simulink model "model"  (R2022b)
settings: Solver=VariableStepAuto  StartTime=0.0  StopTime=3  FixedStep=Tsi/10  RelTol=2e-4
undefined symbols (not defined in the file): B, B0, Hpp, Imax, In, Kdp_si, Ke, Kf, Ki_si, Kip_si, Kp_si, Kpp_si, Kppph_si, Kpppl_si, L, M, max_ppa_si, max_ppv_si, R, Umax
libraries: simulink x3, slctrlblks x1
settings Model: Creator=Giulio  LastModifiedBy=niczan1
settings DebuggingCC: UnconnectedInputMsg=warning  UnconnectedOutputMsg=warning  UnconnectedLineMsg=warning  SFMachineParentedDataDiag=warning
settings ModelReferenceCC: EnableRefExpFcnMdlSchedulingChecks=on

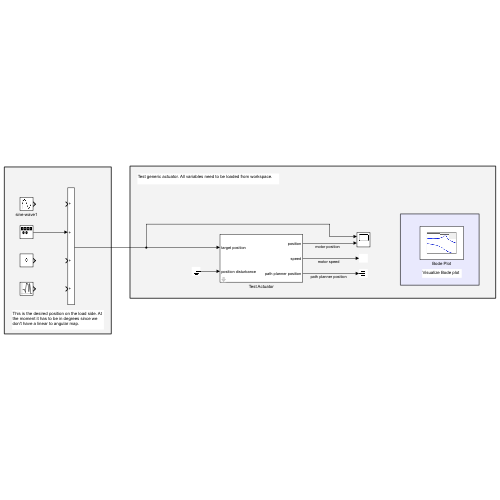
[thumbnail: Simulink's stored preview of the top-level diagram]
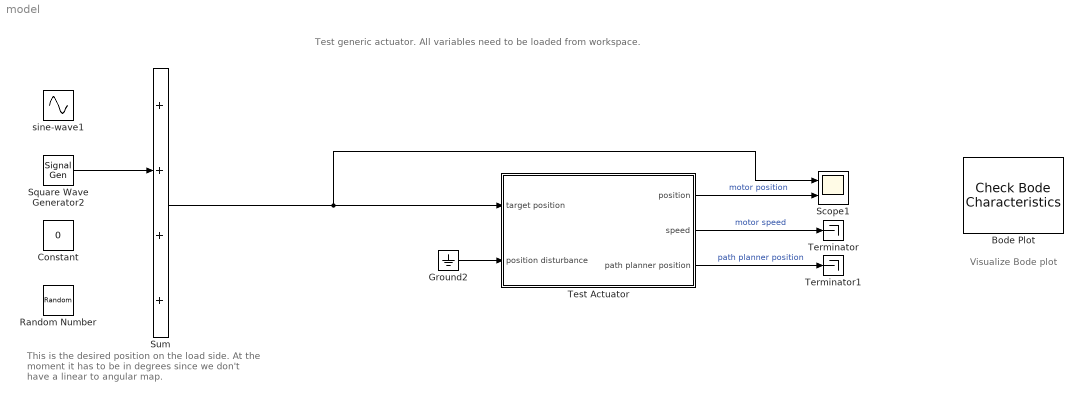
== system model ==
  note: This is the desired position on the load side. At the moment it has to be in degrees since we don't have a linear to angular map.
  note: Visualize Bode plot
  note: Test generic actuator. All variables need to be loaded from workspace.
  Bode Plot : slctrlblks/Model Verification/Check Bode  Characteristics  InstantiateOnLoad=on  SaveOperatingPoints=off  LinearizationIOs={'/Sum', 1, 'in', 'off', '';'/Test Actuator', 1, 'out', 'on', ''}  LinearizeAt=SnapshotTimes  SnapshotTimes=[0]  TriggerType=rising  SampleTime=auto  RateConversionMethod=zoh  PreWarpFreq=10  UseExactDelayModel=off  UseFullBlockNameLabels=off  UseBusSignalLabels=off  enabled=on  stopWhenAssertionFail=off  export=off  ViewDlgPos=[2544 169 510 390]  OpenViewOnLoad=off  LaunchViewOnOpen=on  FrequencyUnits=rad/s  MagnitudeUnits=dB  PhaseUnits=deg  TimeUnits=seconds  EnableUpperBound=off  UpperBoundFrequencies=[]  UpperBoundMagnitudes=[]  EnableLowerBound=off  LowerBoundFrequencies=[]  LowerBoundMagnitudes=[]
      settings: LibrarySourceBlock=slctrlblks/Linear Analysis Plots/Bode Plot
  Constant : Constant  Value=0
  Ground2 : Ground
  Random Number : RandomNumber  Variance=1e-10  SampleTime=1e-3
  Scope1 : Scope  NumInputPorts=2
  Square Wave Generator2 : SignalGenerator  WaveForm=square  Amplitude=15e-3
  Sum : Sum  Inputs=++++
  Terminator : Terminator
  Terminator1 : Terminator
  Test Actuator : Subsystem  mask(Motor servo){Tsi=4e-5, Tsp=4e-4, Tspp=4e-4}
      mask DialogControl SamplingTimes Prompt: Sampling times
  sine-wave1 : Sin  Amplitude=2.5e-3  Frequency=2*pi*4  SampleTime=0
  wires:
  Sum/1 -> Test Actuator/1(target position), Scope1/1
  Test Actuator/3(path planner position) -> Terminator1/1  "path planner position"
  Test Actuator/2(speed) -> Terminator/1  "motor speed"
  Ground2/1 -> Test Actuator/2(position disturbance)
  Square Wave Generator2/1 -> Sum/2
  Test Actuator/1(position) -> Scope1/2  "motor position"

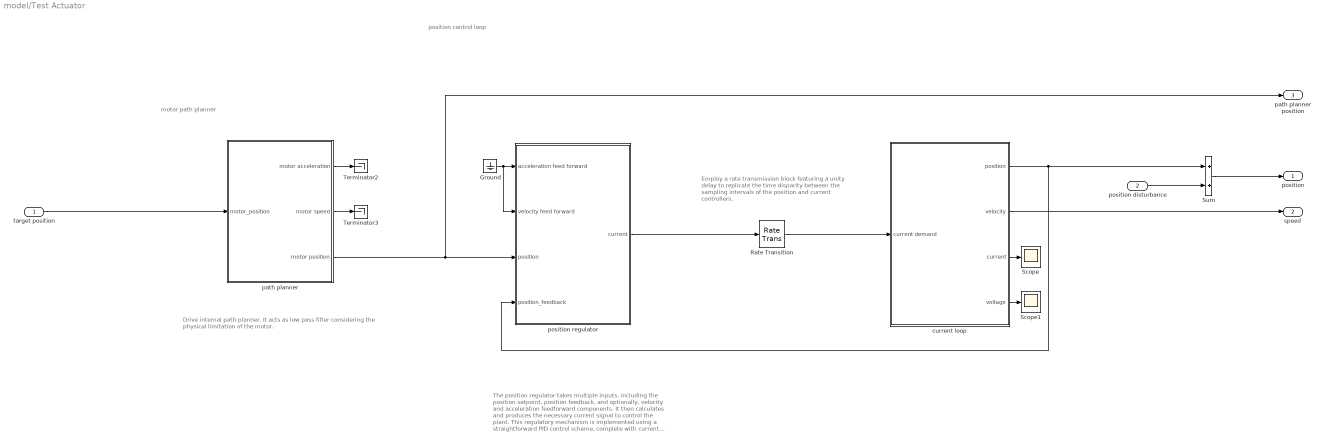
== system model/Test Actuator ==
  note: position control loop
  note: Employ a rate transmission block featuring a unity delay to replicate the time disparity between the sampling intervals of the position and current controllers.
  note: The position regulator takes multiple inputs, including the position setpoint, position feedback, and optionally, velocity and acceleration feedforward components. It then calculates and produces the necessary current signal to control the plant. This regulatory mechanism is implemented using a straightforward PID control scheme, complete with current saturation (limited to the motor's nominal current) and anti-windup provisions.
  note: motor path planner
  note: Drive internal path planner. It acts as low pass filter considering the physical limitation of the motor.
  target position : Inport
  position disturbance : Inport  Port=2
  Ground : Ground
  Rate Transition : RateTransition
  Scope : Scope
  Scope1 : Scope
  Sum : Sum
  Terminator2 : Terminator
  Terminator3 : Terminator
  current loop : Subsystem
  path planner : Subsystem  TreatAsAtomicUnit=on  SystemSampleTime=Tspp  mask(Drive internal path planner){Active=off, max_ppa_si=max_ppa_si, max_ppv_si=max_ppv_si, Kppph_si=Kppph_si, Kpppl_si=Kpppl_si, Hpp=Hpp}
      mask prompts: max_ppa_si "Max acceleration"; max_ppv_si "Max speed"; Kppph_si "High gain"; Kpppl_si "Low gain"; Hpp "Exponential"
      mask DialogControl ParameterGroupVar Prompt: Status
      mask DialogControl Container3 Prompt: Saturation
      mask DialogControl Container4 Prompt: Controller
  position regulator : Subsystem  TreatAsAtomicUnit=on  SystemSampleTime=Tsp  mask(Position PID controller){In=In, Imax=Imax, Kpp_si=Kpp_si, Kip_si=Kip_si, Kdp_si=Kdp_si, FF_w_si=0, FF_a_si=0}
      mask prompts: In "Nominal current"; Imax "Max current"; Kpp_si "Proportional gain"; Kip_si "Integral gain"; Kdp_si "Derivative gain"; FF_w_si "Velocity feed forward gain"; FF_a_si "Acceleration feed forward gain"
      mask DialogControl Saturation Prompt: Saturation
      mask DialogControl Controller Prompt: Controller
  position : Outport
  speed : Outport  Port=2
  path planner position : Outport  Port=3
  wires:
  position regulator/1(current) -> Rate Transition/1
  current loop/1(position) -> Sum/1, position regulator/4(position_feedback)
  Rate Transition/1 -> current loop/1(current demand)
  current loop/4(voltage) -> Scope1/1
  current loop/3(current) -> Scope/1
  path planner/2(motor speed) -> Terminator3/1
  path planner/1(motor acceleration) -> Terminator2/1
  Ground/1 -> position regulator/2(velocity feed forward), position regulator/1(acceleration feed forward)
  target position/1 -> path planner/1(motor_position)
  current loop/2(velocity) -> speed/1
  position disturbance/1 -> Sum/2
  Sum/1 -> position/1
  path planner/3(motor position) -> path planner position/1, position regulator/3(position)

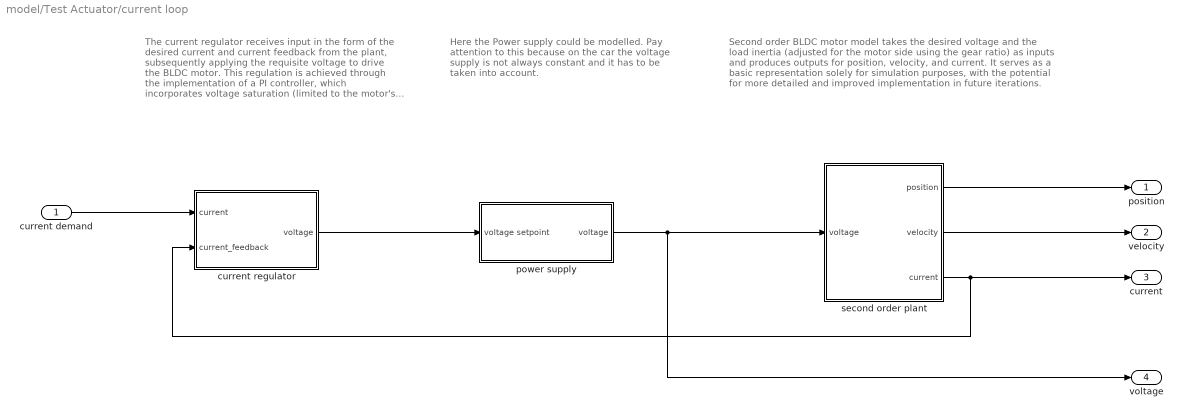
== system model/Test Actuator/current loop ==
  note: The current regulator receives input in the form of the desired current and current feedback from the plant, subsequently applying the requisite voltage to drive the BLDC motor. This regulation is achieved through the implementation of a PI controller, which incorporates voltage saturation (limited to the motor's nominal voltage) and anti-windup mechanisms.
  note: Second order BLDC motor model takes the desired voltage and the load inertia (adjusted for the motor side using the gear ratio) as inputs and produces outputs for position, velocity, and current. It serves as a basic representation solely for simulation purposes, with the potential for more detailed and improved implementation in future iterations.
  note: Here the Power supply could be modelled. Pay attention to this because on the car the voltage supply is not always constant and it has to be taken into account.
  current demand : Inport
  current regulator : Subsystem  TreatAsAtomicUnit=on  SystemSampleTime=Tsi  mask(Current PI controller){Umax=Umax, Un=Umax, Kp_si=Kp_si, Ki_si=Ki_si}
      mask prompts: Umax "Max voltage"; Un "Nominal voltage"; Kp_si "Proportional gain"; Ki_si "Integral gain"
      mask DialogControl Saturation Prompt: Saturation
      mask DialogControl Controller Prompt: Controller
  power supply : Subsystem
  second order plant : Subsystem  mask(Motor second order model){Ke=Ke, R=R, L=L, Kf=Kf, M=M, B=B, B0=B0}
      mask prompts: Ke "Electrical constant"; R "Resistance"; L "Inductance"; Kf "Force constant"; M "Motor mass"; B "Viscous friction"; B0 "Static friction"
      mask DialogControl electrical Prompt: Electrical
      mask DialogControl Mechanical Prompt: Mechanical
  position : Outport
  velocity : Outport  Port=2
  current : Outport  Port=3
  voltage : Outport  Port=4
  wires:
  second order plant/2(velocity) -> velocity/1
  current demand/1 -> current regulator/1(current)
  second order plant/1(position) -> position/1
  second order plant/3(current) -> current regulator/2(current_feedback), current/1
  power supply/1(voltage) -> second order plant/1(voltage), voltage/1
  current regulator/1(voltage) -> power supply/1(voltage setpoint)

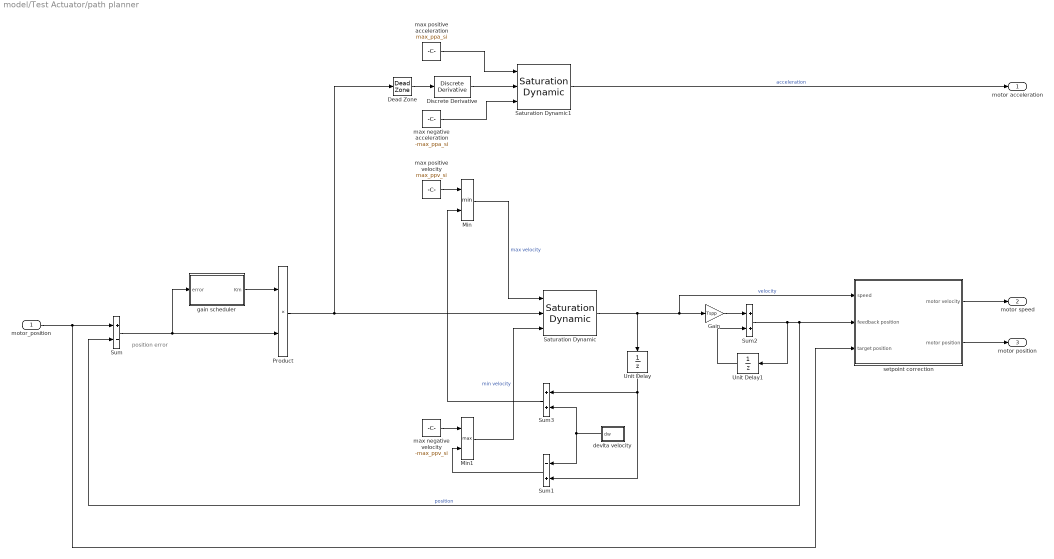
== system model/Test Actuator/path planner ==
  note: position error
  motor_position : Inport
  Dead Zone : DeadZone  LowerValue=-0.01  UpperValue=0.01
  Discrete Derivative : simulink/Discrete/Discrete Derivative  gainval=1.0  ICPrevScaledInput=0.0  OutMin=[]  OutMax=[]  OutDataType=fixdt(1, 16)  OutScaling=2^-10  DoSatur=off
  Gain : Gain  Gain=Tspp
  Min : MinMax  Inputs=2
  Min1 : MinMax  Function=max  Inputs=2
  Product : Product
  Saturation Dynamic : simulink/Discontinuities/Saturation Dynamic  OutMin=[]  OutMax=[]  OutDataTypeStr=Inherit: Same as second input  OutDataType=fixdt(1, 16)  OutScaling=2^-10  DoSatur=off
  Saturation Dynamic1 : simulink/Discontinuities/Saturation Dynamic  OutMin=[]  OutMax=[]  OutDataTypeStr=Inherit: Same as second input  OutDataType=fixdt(1, 16)  OutScaling=2^-10  DoSatur=off
  Sum : Sum  Inputs=+-
  Sum1 : Sum  Inputs=-+
  Sum2 : Sum
  Sum3 : Sum
  Unit Delay : UnitDelay  SampleTime=-1  HasFrameUpgradeWarning=on
  Unit Delay1 : UnitDelay  SampleTime=-1  HasFrameUpgradeWarning=on
  devlta velocity : Subsystem
  gain scheduler : Subsystem
  max negative acceleration : Constant  Value=-max_ppa_si
  max negative velocity : Constant  Value=-max_ppv_si
  max positive acceleration : Constant  Value=max_ppa_si
  max positive velocity : Constant  Value=max_ppv_si
  setpoint correction : Subsystem
  motor acceleration : Outport
  motor speed : Outport  Port=2
  motor position : Outport  Port=3
  wires:
  Sum/1 -> gain scheduler/1(error), Product/2
  max positive velocity/1 -> Min/1
  Saturation Dynamic/1 -> Gain/1, setpoint correction/1(speed), Unit Delay/1  "velocity"
  devlta velocity/1(dw) -> Sum1/1, Sum3/2
  Sum3/1 -> Min/2
  max negative velocity/1 -> Min1/1
  Sum1/1 -> Min1/2
  Min1/1 -> Saturation Dynamic/3  "min velocity"
  Min/1 -> Saturation Dynamic/1  "max velocity"
  Sum2/1 -> setpoint correction/2(feedback position), Sum/2, Unit Delay1/1  "position"
  Unit Delay/1 -> Sum3/1, Sum1/2
  max positive acceleration/1 -> Saturation Dynamic1/1
  max negative acceleration/1 -> Saturation Dynamic1/3
  Saturation Dynamic1/1 -> motor acceleration/1  "acceleration"
  Discrete Derivative/1 -> Saturation Dynamic1/2
  Dead Zone/1 -> Discrete Derivative/1
  setpoint correction/1(motor velocity) -> motor speed/1
  gain scheduler/1(Km) -> Product/1
  motor_position/1 -> setpoint correction/3(target position), Sum/1
  setpoint correction/2(motor position) -> motor position/1
  Product/1 -> Dead Zone/1, Saturation Dynamic/2
  Gain/1 -> Sum2/1
  Unit Delay1/1 -> Sum2/2

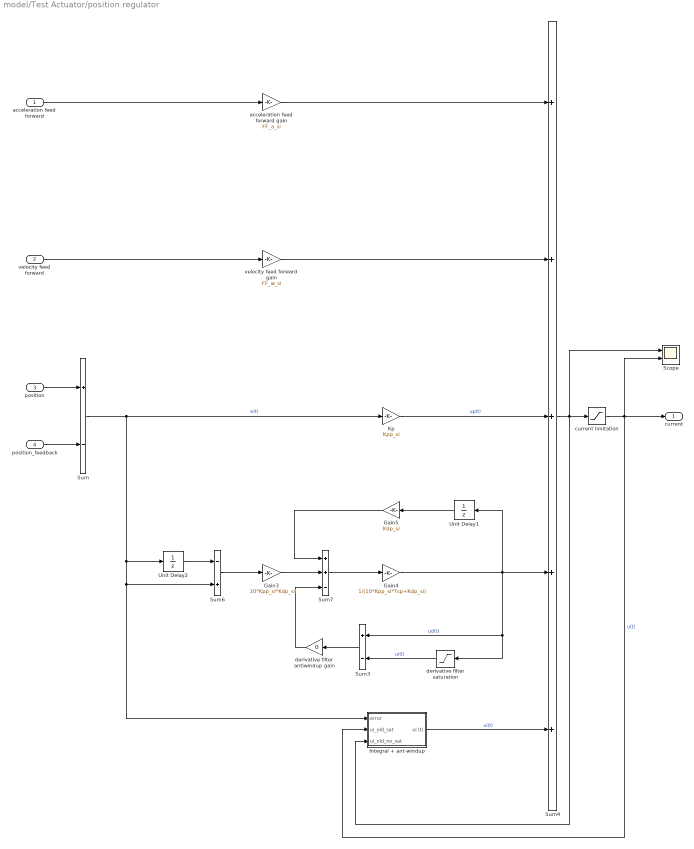
== system model/Test Actuator/position regulator ==
  acceleration feed forward : Inport
  velocity feed forward : Inport  Port=2
  position : Inport  Port=3
  position_feedback : Inport  Port=4
  Gain3 : Gain  Gain=10*Kpp_si*Kdp_si
  Gain4 : Gain  Gain=1/(10*Kpp_si*Tsp+Kdp_si)
  Gain5 : Gain  Gain=Kdp_si
  Integral + ant-windup : Subsystem
  Kp : Gain  Gain=Kpp_si
  Scope : Scope  NumInputPorts=2
  Sum : Sum  Inputs=+-
  Sum3 : Sum  Inputs=+-
  Sum4 : Sum  Inputs=+++++
  Sum6 : Sum  Inputs=-+
  Sum7 : Sum  Inputs=++-
  Unit Delay1 : UnitDelay  SampleTime=-1  HasFrameUpgradeWarning=on
  Unit Delay2 : UnitDelay  SampleTime=-1  HasFrameUpgradeWarning=on
  acceleration feed forward gain : Gain  Gain=FF_a_si
  current limitation : Saturate  UpperLimit=Imax  LowerLimit=-Imax
  derivative filter antiwindup gain : Gain  Gain=0
  derivative filter saturation : Saturate  UpperLimit=Imax/2  LowerLimit=-Imax/2
  velocity feed forward gain : Gain  Gain=FF_w_si
  current : Outport
  wires:
  acceleration feed forward gain/1 -> Sum4/1
  acceleration feed forward/1 -> acceleration feed forward gain/1
  velocity feed forward gain/1 -> Sum4/2
  velocity feed forward/1 -> velocity feed forward gain/1
  Sum7/1 -> Gain4/1
  current limitation/1 -> current/1, Scope/2, Integral + ant-windup/2(ui_old_sat)  "u(t)"
  Unit Delay2/1 -> Sum6/1
  Sum6/1 -> Gain3/1
  Unit Delay1/1 -> Gain5/1
  Kp/1 -> Sum4/3  "up(t)"
  Sum/1 -> Kp/1, Integral + ant-windup/1(error), Sum6/2, Unit Delay2/1  "e(t)"
  Gain3/1 -> Sum7/2
  Gain5/1 -> Sum7/1
  Gain4/1 -> Sum4/4, derivative filter saturation/1, Sum3/1, Unit Delay1/1  "ud(t)"
  Sum3/1 -> derivative filter antiwindup gain/1
  derivative filter saturation/1 -> Sum3/2  "ui(t)"
  derivative filter antiwindup gain/1 -> Sum7/3
  Integral + ant-windup/1(ui (t)) -> Sum4/5  "ui(t)"
  Sum4/1 -> Scope/1, current limitation/1, Integral + ant-windup/3(ui_old_no_sat)
  position/1 -> Sum/1
  position_feedback/1 -> Sum/2

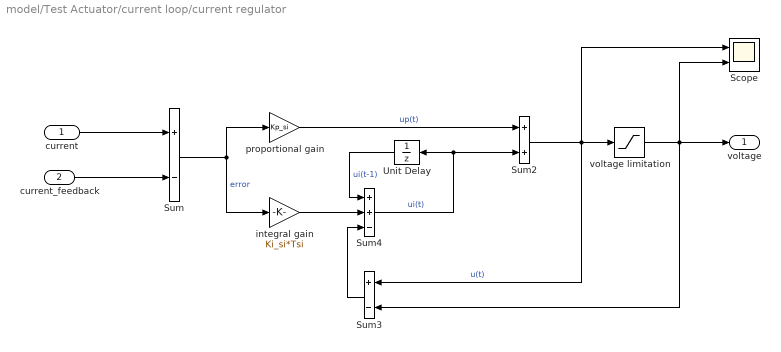
== system model/Test Actuator/current loop/current regulator ==
  current : Inport
  current_feedback : Inport  Port=2
  Scope : Scope  NumInputPorts=2
  Sum : Sum  Inputs=+-
  Sum2 : Sum
  Sum3 : Sum  Inputs=+-
  Sum4 : Sum  Inputs=++-
  Unit Delay : UnitDelay  SampleTime=-1  HasFrameUpgradeWarning=on
  integral gain : Gain  Gain=Ki_si*Tsi
  proportional gain : Gain  Gain=Kp_si
  voltage limitation : Saturate  UpperLimit=Umax  LowerLimit=-Umax
  voltage : Outport
  wires:
  voltage limitation/1 -> Scope/2, voltage/1, Sum3/2
  Sum3/1 -> Sum4/3
  Sum4/1 -> Unit Delay/1, Sum2/2  "ui(t)"
  Sum2/1 -> Sum3/1, Scope/1, voltage limitation/1  "u(t)"
  Sum/1 -> integral gain/1, proportional gain/1  "error"
  proportional gain/1 -> Sum2/1  "up(t)"
  current/1 -> Sum/1
  current_feedback/1 -> Sum/2
  Unit Delay/1 -> Sum4/1  "ui(t-1)"
  integral gain/1 -> Sum4/2

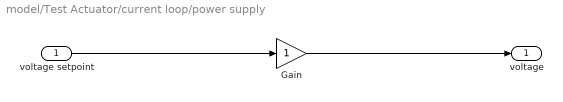
== system model/Test Actuator/current loop/power supply ==
  voltage setpoint : Inport
  Gain : Gain
  voltage : Outport
  wires:
  Gain/1 -> voltage/1
  voltage setpoint/1 -> Gain/1

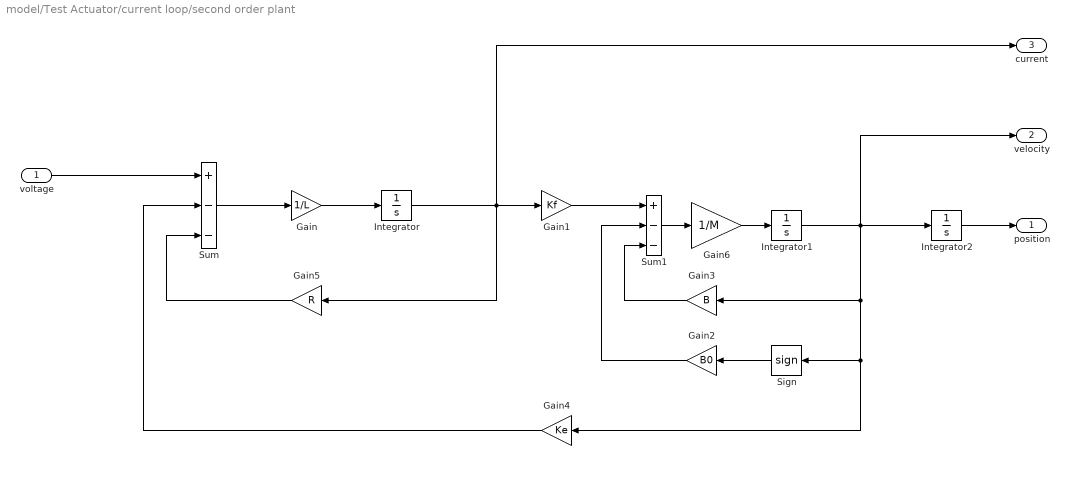
== system model/Test Actuator/current loop/second order plant ==
  voltage : Inport
  Gain : Gain  Gain=1/L
  Gain1 : Gain  Gain=Kf
  Gain2 : Gain  Gain=B0
  Gain3 : Gain  Gain=B
  Gain4 : Gain  Gain=Ke
  Gain5 : Gain  Gain=R
  Gain6 : Gain  Gain=1/M
  Integrator : Integrator
  Integrator1 : Integrator
  Integrator2 : Integrator
  Sign : Signum
  Sum : Sum  Inputs=+--
  Sum1 : Sum  Inputs=+--
  position : Outport
  velocity : Outport  Port=2
  current : Outport  Port=3
  wires:
  Integrator2/1 -> position/1
  voltage/1 -> Sum/1
  Gain/1 -> Integrator/1
  Sum1/1 -> Gain6/1
  Gain5/1 -> Sum/3
  Gain6/1 -> Integrator1/1
  Gain4/1 -> Sum/2
  Sum/1 -> Gain/1
  Gain1/1 -> Sum1/1
  Sign/1 -> Gain2/1
  Gain3/1 -> Sum1/3
  Gain2/1 -> Sum1/2
  Integrator/1 -> current/1, Gain5/1, Gain1/1
  Integrator1/1 -> velocity/1, Integrator2/1, Sign/1, Gain4/1, Gain3/1

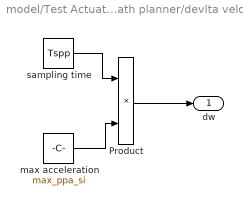
== system model/Test Actuator/path planner/devlta velocity ==
  Product : Product
  max acceleration : Constant  Value=max_ppa_si
  sampling time : Constant  Value=Tspp
  dw : Outport
  wires:
  sampling time/1 -> Product/1
  Product/1 -> dw/1
  max acceleration/1 -> Product/2

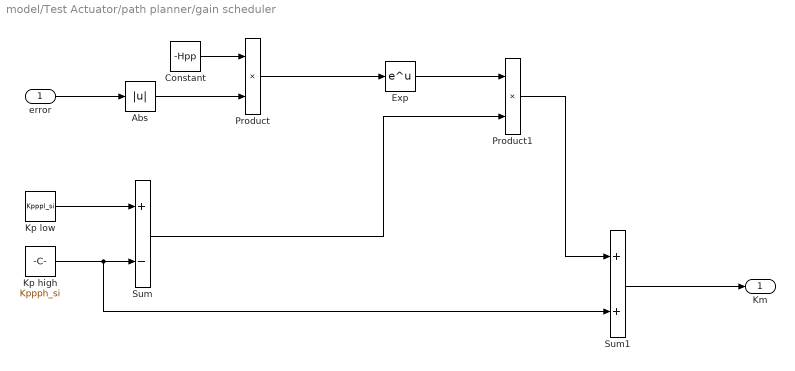
== system model/Test Actuator/path planner/gain scheduler ==
  error : Inport
  Abs : Abs  SaturateOnIntegerOverflow=off
  Constant : Constant  Value=-Hpp
  Exp : Math
  Kp high : Constant  Value=Kppph_si
  Kp low : Constant  Value=Kpppl_si
  Product : Product
  Product1 : Product
  Sum : Sum  Inputs=+-
  Sum1 : Sum
  Km : Outport
  wires:
  Constant/1 -> Product/1
  Product/1 -> Exp/1
  Exp/1 -> Product1/1
  Abs/1 -> Product/2
  Kp low/1 -> Sum/1
  Kp high/1 -> Sum1/2, Sum/2
  Sum/1 -> Product1/2
  Product1/1 -> Sum1/1
  error/1 -> Abs/1
  Sum1/1 -> Km/1

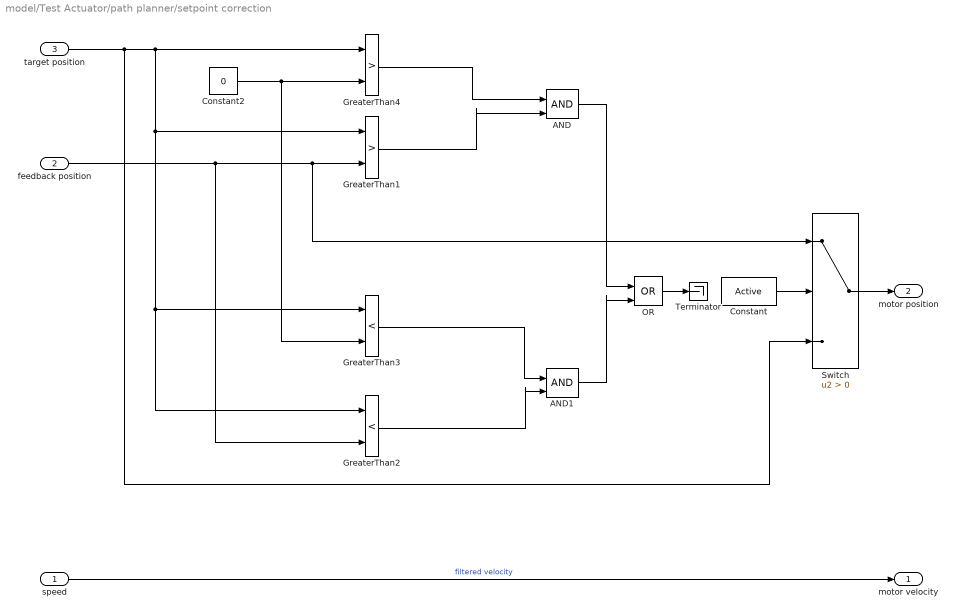
== system model/Test Actuator/path planner/setpoint correction ==
  speed : Inport
  feedback position : Inport  Port=2
  target position : Inport  Port=3
  AND : Logic  IconShape=distinctive  AllPortsSameDT=off  OutDataTypeStr=boolean
  AND1 : Logic  IconShape=distinctive  AllPortsSameDT=off  OutDataTypeStr=boolean
  Constant : Constant  Value=Active  OutDataTypeStr=boolean
  Constant2 : Constant  Value=0
  GreaterThan1 : RelationalOperator  Operator=>  OutDataTypeStr=boolean  RndMeth=Simplest  InputSameDT=off
  GreaterThan2 : RelationalOperator  Operator=<  OutDataTypeStr=boolean  RndMeth=Simplest  InputSameDT=off
  GreaterThan3 : RelationalOperator  Operator=<  OutDataTypeStr=boolean  RndMeth=Simplest  InputSameDT=off
  GreaterThan4 : RelationalOperator  Operator=>  OutDataTypeStr=boolean  RndMeth=Simplest  InputSameDT=off
  OR : Logic  Operator=OR  IconShape=distinctive  AllPortsSameDT=off  OutDataTypeStr=boolean
  Switch : Switch  Criteria=u2 > Threshold  SaturateOnIntegerOverflow=off  InputSameDT=off
  Terminator : Terminator
  motor velocity : Outport
  motor position : Outport  Port=2
  wires:
  GreaterThan3/1 -> AND1/1
  GreaterThan1/1 -> AND/2
  GreaterThan4/1 -> AND/1
  AND1/1 -> OR/2
  AND/1 -> OR/1
  Switch/1 -> motor position/1
  GreaterThan2/1 -> AND1/2
  speed/1 -> motor velocity/1  "filtered velocity"
  feedback position/1 -> GreaterThan2/2, Switch/1, GreaterThan1/2
  Constant2/1 -> GreaterThan3/2, GreaterThan4/2
  Constant/1 -> Switch/2
  OR/1 -> Terminator/1
  target position/1 -> Switch/3, GreaterThan3/1, GreaterThan2/1, GreaterThan1/1, GreaterThan4/1

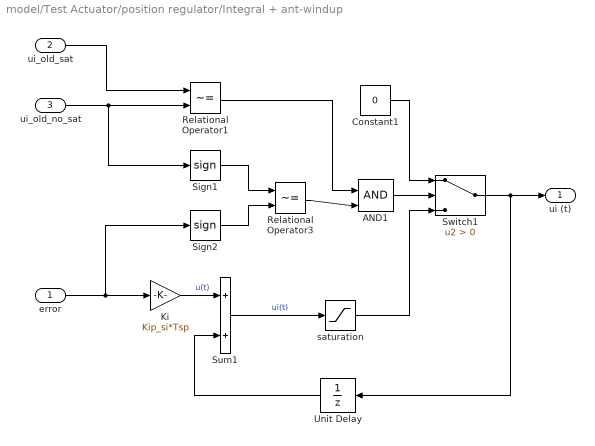
== system model/Test Actuator/position regulator/Integral + ant-windup ==
  error : Inport
  ui_old_sat : Inport  Port=2
  ui_old_no_sat : Inport  Port=3
  AND1 : Logic  IconShape=distinctive  AllPortsSameDT=off  OutDataTypeStr=boolean
  Constant1 : Constant  Value=0
  Ki : Gain  Gain=Kip_si*Tsp
  Relational Operator1 : RelationalOperator  Operator=~=  OutDataTypeStr=boolean  RndMeth=Simplest  InputSameDT=off
  Relational Operator3 : RelationalOperator  Operator=~=  OutDataTypeStr=boolean  RndMeth=Simplest  InputSameDT=off
  Sign1 : Signum
  Sign2 : Signum
  Sum1 : Sum
  Switch1 : Switch  Criteria=u2 > Threshold  SaturateOnIntegerOverflow=off  InputSameDT=off
  Unit Delay : UnitDelay  SampleTime=-1  HasFrameUpgradeWarning=on
  saturation : Saturate  UpperLimit=In  LowerLimit=-In
  ui (t) : Outport
  wires:
  Sign2/1 -> Relational Operator3/2
  error/1 -> Ki/1, Sign2/1
  Constant1/1 -> Switch1/1
  ui_old_sat/1 -> Relational Operator1/1
  ui_old_no_sat/1 -> Sign1/1, Relational Operator1/2
  Relational Operator3/1 -> AND1/2
  Relational Operator1/1 -> AND1/1
  Sign1/1 -> Relational Operator3/1
  AND1/1 -> Switch1/2
  Switch1/1 -> ui (t)/1, Unit Delay/1
  Sum1/1 -> saturation/1  "ui(t)"
  Ki/1 -> Sum1/1  "u(t)"
  Unit Delay/1 -> Sum1/2
  saturation/1 -> Switch1/3
